simulink model "QBot2_TRIAL_1"  (Simulink 8.6)
settings: Solver=ode1  StartTime=0.0  StopTime=inf  FixedStep=0.01  RelTol=1e-3
undefined symbols (not defined in the file): HIL, Kinect, qc_get_step_size
libraries: quarc_library x13, simulink x1
settings Model: Creator=drmadill  LastModifiedBy=rclue  SimulationMode=external  ExtModeTrigDuration=1
settings SolverCC: PositivePriorityOrder=on
settings DebuggingCC: FcnCallInpInsideContextMsg=UseLocalSettings
settings RTWCC: SystemTargetFile=quarc_linux_duovero.tlc  TemplateMakefile=quarc_linux_duovero_tmf  Description=QUARC Linux DuoVero Target
settings STFCustomTargetCC: TargetLibSuffix=.a  TargetPreCompLibLocation=C:\PROGRA~3\QUARC\lib\2015b\LINUX_~1\release  ConcurrentExecutionCompliant=on  GeneratePreprocessorConditionals=Disable all  CPPClassGenCompliant=on  SystemTargetFile=quarc_linux_duovero.tlc
settings GRTTargetCC: TargetLibSuffix=.a  TargetPreCompLibLocation=C:\PROGRA~3\QUARC\lib\2015b\LINUX_~1\release  ParMdlRefBuildCompliant=off  CompOptLevelCompliant=off  MatFileLogging=off  UseToolchainInfoCompliant=off  ExtMode=on  ExtModeMexFile=quarc_comm  ExtModeMexArgs='-w -d /tmp -uri %u', 'tcpip://192.168.2.49:17001'

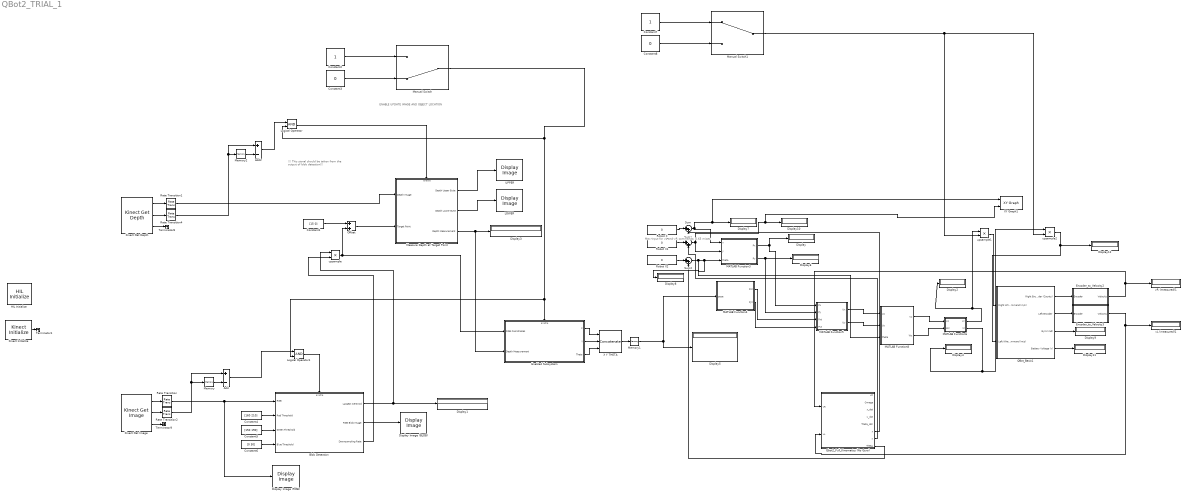
== system QBot2_TRIAL_1 ==
  note: ENABLE UPDATE IMAGE AND OBJECT LOCATION
  note: !!! This signal should be taken from the output of blob detection!!!
  note: Max input for vL and vR commands: 0.65 m/sec
  Add : Sum  Inputs=+-
  Add2 : Sum  Inputs=+-
  Blob Detection : Subsystem  TreatAsAtomicUnit=on
  Constant1 : Constant  Value=[15 0]
  Constant2 : Constant
  Constant3 : Constant  Value=0
  Constant4 : Constant  Value=[160 210]
  Constant5 : Constant  Value=[150 190]
  Constant6 : Constant  Value=[0 30]
  Constant7 : Constant
  Constant8 : Constant  Value=0
  Display{,1..12} (13 alike) : Display
  Display Image (BLOB) : quarc_library/Sinks/Figures/Display Image  figure_mode=Use figure window  figure_tag=figure1  axes_tag=axes1  update_rate=1  initial_position="167  215  854  628"  initial_visibility=off  sample_time=-1  axes_only=off  orig_size=off
  Display Image (RGB) : quarc_library/Sinks/Figures/Display Image  figure_mode=Use figure window  figure_tag=figure1  axes_tag=axes1  update_rate=1  initial_position="328  208  854  628"  initial_visibility=off  sample_time=-1  axes_only=off  orig_size=off
  Enabled Subsystem : Subsystem  TreatAsAtomicUnit=on
  Encoder_to_Velocity2 : Subsystem
  Encoder_to_Velocity3 : Subsystem
  HIL Initialize : quarc_library/Data Acquisition/Generic/Configuration/HIL Initialize  Priority=-99  object_name=HIL-1  board_type=qbot2  board_number=0  board_options=enc0_dir=0;enc0_filter=1;enc0_a=0;enc0_b=0;enc0_z=1;enc0_reload=0;enc1_dir=0;enc1_filter=1;enc1_a=0;enc1_b=0;enc1_z=1;enc1_reload=0;pwm0_immediate=0;pwm1_immediate=0;pwm2_immediate=0;pwm3_immediate=0;  exclusive=off  active=off  hardware_clocks=[]  clock_modes=[]  initial_clock_frequencies=[]  set_clock_params_at_start=off  set_clock_params_at_switch_in=off  set_clock_frequencies_at_start=off  set_clock_frequencies_at_switch_in=off  analog_input_channels=[0:9]  analog_input_maximums=[5 5 5 5 16.5 3.3 3.3 3.3 3.3]  analog_input_minimums=[0 0 0 0 0 0 0 0 0]  set_analog_input_params_at_start=off  set_analog_input_params_at_switch_in=off  analog_output_channels=[]  analog_output_maximums=[]  analog_output_minimums=[]  initial_analog_outputs=[]  final_analog_outputs=[]  watchdog_analog_outputs=[]  set_analog_output_params_at_start=off  set_analog_output_params_at_switch_in=off  set_analog_outputs_at_start=off  set_analog_outputs_at_switch_in=off  set_analog_outputs_at_terminate=off  set_analog_outputs_at_switch_out=off  set_analog_outputs_on_watchdog=off  digital_input_channels=[]  digital_output_channels=[]  digital_output_configuration=[]  initial_digital_outputs=[0]  final_digital_outputs=[0]  watchdog_digital_outputs=[0]  set_digital_output_params_at_start=off  set_digital_output_params_at_switch_in=off  set_digital_outputs_at_start=on  set_digital_outputs_at_switch_in=off  set_digital_outputs_at_terminate=on  set_digital_outputs_at_switch_out=off  set_digital_outputs_on_watchdog=on  encoder_channels=[0:3]  quadrature=[4]  encoder_filter_frequency=[]  initial_encoder_counts=[0]  set_encoder_params_at_start=on  set_encoder_params_at_switch_in=off  set_encoder_counts_at_start=on  set_encoder_counts_at_switch_in=off  pwm_channels=[0:3]  pwm_modes=[0]  pwm_frequency=[20e6/1024]  pwm_configuration=[0]  pwm_alignment=[0]  pwm_polarity=[1]  pwm_leading_deadband=[0]  pwm_trailing_deadband=[0]  initial_pwm_outputs=[0]  final_pwm_outputs=[0]  watchdog_pwm_outputs=[0]  set_pwm_params_at_start=on  set_pwm_params_at_switch_in=off  set_pwm_outputs_at_start=on  set_pwm_outputs_at_switch_in=off  set_pwm_outputs_at_terminate=on  set_pwm_outputs_at_switch_out=off  set_pwm_outputs_on_watchdog=on  other_output_channels=[2000:2001 14000 16000]  initial_other_outputs=[0 0 0 7]  final_other_outputs=[0 0 0 7]  watchdog_other_outputs=[]  set_other_outputs_at_start=on  set_other_outputs_at_switch_in=off  set_other_outputs_at_terminate=on  set_other_outputs_at_switch_out=off  set_other_outputs_on_watchdog=off
  Kinect Get Depth : quarc_library/Multimedia/Kinect Get Depth  object_name=Kinect-1  resolution=640 x 480  sample_time=qc_get_step_size * ceil(0.1 / qc_get_step_size)  show_player=off
  Kinect Get Image : quarc_library/Multimedia/Kinect Get Image  object_name=Kinect-1  sensor_type=color  resolution=640 x 480  output_format=MATLAB RGB (HxWx3)  data_type=uint8  backlight=average brightness  flicker=none  brightness=0.2156  gain=1.0  gamma=2.2  autoexposure=on  exposure=0  contrast=1.0  sharpness=0.5  hue=0.0  saturation=1.0  autobalance=on  balance=2700  frame_interval=0  sample_time=qc_get_step_size * ceil(0.1 / qc_get_step_size)
  Kinect Initialize : quarc_library/Multimedia/Kinect Initialize  object_name=Kinect-1  kinect_type=Kinect for XBox 360  identifier=0  sample_time=qc_get_step_size * ceil(0.033 / qc_get_step_size)  active=on
  LOWER : quarc_library/Sinks/Figures/Display Image  figure_mode=Use figure window  figure_tag=figure1  axes_tag=axes1  update_rate=1  initial_position="340  252  854  628"  initial_visibility=off  sample_time=-1  axes_only=off  orig_size=off
  Logical Operator : Logic  AllPortsSameDT=off  OutDataTypeStr=boolean
  Logical Operator1 : Logic  AllPortsSameDT=off  OutDataTypeStr=boolean
  MATLAB Function3 : MATLAB Function  TreatAsAtomicUnit=on
  MATLAB Function4 : MATLAB Function  TreatAsAtomicUnit=on
  MATLAB Function5 : MATLAB Function  TreatAsAtomicUnit=on
  MATLAB Function6 : MATLAB Function  TreatAsAtomicUnit=on
  MATLAB Function8 : MATLAB Function  TreatAsAtomicUnit=on
  Manual Switch : ManualSwitch  CurrentSetting=0
  Manual Switch1 : ManualSwitch
  Measure Depth at Target Point : Subsystem  TreatAsAtomicUnit=on
  Memory : Memory
  Memory1 : Memory
  Memory2 : Memory
  Offset : Sum
  QBot_Basic1 : Subsystem
  Qbot2_Full_Kinematics (No Gyro) : Subsystem
  Rate Transition{,1..2,4} (4 alike) : RateTransition
  Robot X : Constant  Value=0
  Robot X1 : Constant  Value=0
  Robot X2 : Constant  Value=0
  Sum : Sum  Inputs=|++
  Sum1 : Sum  Inputs=|++
  Sum2 : Sum  Inputs=|++
  Terminator1 : Terminator
  Terminator8 : Terminator
  Terminator9 : Terminator
  UPPER : quarc_library/Sinks/Figures/Display Image  figure_mode=Use figure window  figure_tag=figure1  axes_tag=axes1  update_rate=1  initial_position="188  236  854  628"  initial_visibility=off  sample_time=-1  axes_only=off  orig_size=off
  X Y THETA : Concatenate  NumInputs=3  ConcatenateDimension=3
  XY Graph1 : simulink/Sinks/XY Graph  xmin=-3  xmax=3  ymin=-3  ymax=3  st=-1
  upsample : Product
  upsample1 : Product
  upsample2 : Product
  vL (measured)1 : Display
  vR (measured)1 : Display
  wires:
  Kinect Initialize/1 -> Terminator1/1
  Rate Transition4/1 -> Add2/1, Memory2/1
  Memory2/1 -> Add2/2
  Kinect Get Depth/1 -> Rate Transition1/1
  Kinect Get Depth/2 -> Rate Transition4/1
  Kinect Get Depth/3 -> Terminator8/1
  Constant4/1 -> Blob Detection/2(Red Threshold)
  Constant5/1 -> Blob Detection/3(Green Threshold)
  Constant6/1 -> Blob Detection/4(Blue Threshold)
  Kinect Get Image/1 -> Rate Transition/1
  Kinect Get Image/2 -> Rate Transition2/1
  Rate Transition2/1 -> Add/1, Memory/1
  Kinect Get Image/3 -> Terminator9/1
  Rate Transition/1 -> Display Image (RGB)/1, Blob Detection/1(RGB)
  Blob Detection/2(RGB Blob Image) -> Display Image (BLOB)/1
  Rate Transition1/1 -> Measure Depth at Target Point/1(Depth Image)
  Constant1/1 -> Offset/1
  Measure Depth at Target Point/3(Depth Measurement) -> Enabled Subsystem/2(Depth Measurement), Display3/1
  Blob Detection/1(Largest Centroid) -> upsample/1, Display1/1
  Blob Detection/3(Downsampling Rate) -> upsample/2
  Measure Depth at Target Point/1(Depth Upper Byte) -> UPPER/1
  Measure Depth at Target Point/2(Depth Lower Byte) -> LOWER/1
  Offset/1 -> Measure Depth at Target Point/2(Target Point)
  Memory/1 -> Add/2
  MATLAB Function4/1(Pxt) -> MATLAB Function5/3(Pxt)
  MATLAB Function4/2(Pyt) -> MATLAB Function5/4(Pyt)
  MATLAB Function3/2(Py) -> MATLAB Function5/2(Py), Display6/1
  MATLAB Function3/1(Px) -> MATLAB Function5/1(Px), Display/1
  Sum2/1 -> MATLAB Function8/3(theta), Display8/1, MATLAB Function3/3(theta)
  Robot X2/1 -> Sum2/1
  Robot X/1 -> Sum/1
  Robot X1/1 -> Sum1/1
  MATLAB Function5/1(Ux) -> MATLAB Function8/1(Ux)
  MATLAB Function5/2(Uy) -> MATLAB Function8/2(Uy)
  MATLAB Function8/1(Vc) -> MATLAB Function6/1(Vc)
  MATLAB Function8/2(Wc) -> MATLAB Function6/2(Wc)
  MATLAB Function6/1(Vr) -> upsample1/1, Display2/1
  MATLAB Function6/2(Vl) -> Display4/1, upsample2/1
  QBot_Basic1/1(Right Encoder (Counts)) -> Encoder_to_Velocity2/1(Encoder)
  QBot_Basic1/2(Left Encoder) -> Encoder_to_Velocity3/1(Encoder)
  QBot_Basic1/3(Gyro (rad)) -> Display9/1
  QBot_Basic1/4(Battery Voltage (v)) -> Display11/1
  Encoder_to_Velocity2/1(Velocity) -> Qbot2_Full_Kinematics (No Gyro)/1(vR), vR (measured)1/1
  Encoder_to_Velocity3/1(Velocity) -> Qbot2_Full_Kinematics (No Gyro)/2(vL), vL (measured)1/1
  Sum1/1 -> MATLAB Function3/2(y), XY Graph1/2, Display10/1
  Sum/1 -> MATLAB Function3/1(x), XY Graph1/1, Display7/1
  Qbot2_Full_Kinematics (No Gyro)/6(x) -> Sum/2
  Qbot2_Full_Kinematics (No Gyro)/7(y) -> Sum1/2
  Qbot2_Full_Kinematics (No Gyro)/8(Theta) -> Sum2/2
  upsample/1 -> Offset/2, Enabled Subsystem/1(RGB Coordinates)
  Enabled Subsystem/2(Y) -> X Y THETA/2
  Enabled Subsystem/1(X) -> X Y THETA/1
  Enabled Subsystem/3(Theta) -> X Y THETA/3
  Constant3/1 -> Manual Switch/2
  Constant2/1 -> Manual Switch/1
  Manual Switch/1 -> Logical Operator/2, Logical Operator1/2, Enabled Subsystem/Enable
  X Y THETA/1 -> Memory1/1
  Memory1/1 -> MATLAB Function4/1(pose), Display5/1
  upsample1/1 -> QBot_Basic1/1(Right Wheel Command (m/s))
  upsample2/1 -> Display12/1, QBot_Basic1/2(Left Wheel Command (m/s))
  Constant8/1 -> Manual Switch1/2
  Constant7/1 -> Manual Switch1/1
  Manual Switch1/1 -> upsample2/2, upsample1/2
  Add2/1 -> Logical Operator/1
  Add/1 -> Logical Operator1/1
  Logical Operator1/1 -> Blob Detection/Enable
  Logical Operator/1 -> Measure Depth at Target Point/Enable

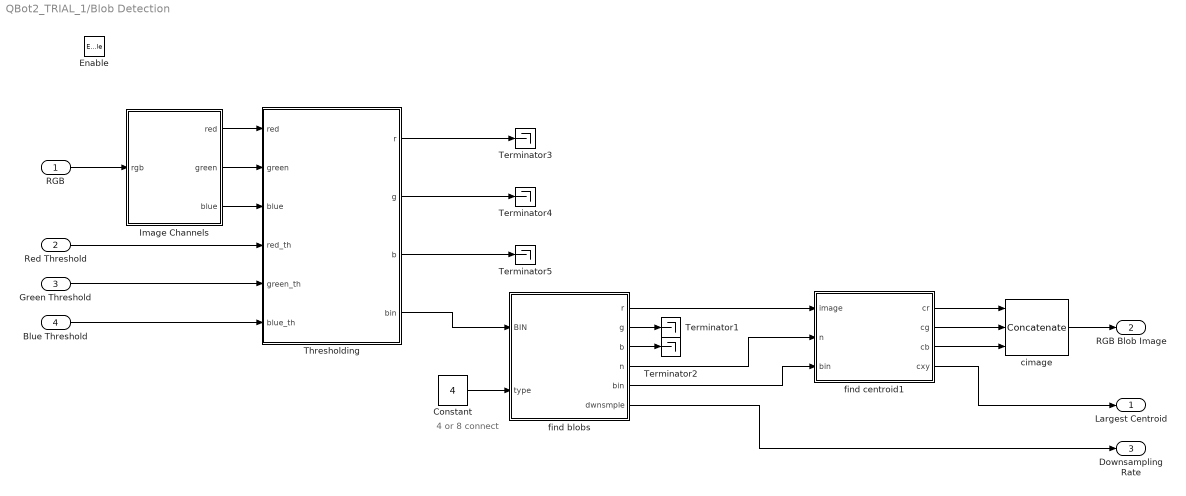
== system QBot2_TRIAL_1/Blob Detection ==
  note: 4 or 8 connect
  RGB : Inport
  Red Threshold : Inport  Port=2
  Green Threshold : Inport  Port=3
  Blue Threshold : Inport  Port=4
  Enable : EnablePort
  Constant : Constant  Value=4
  Image Channels : Subsystem
  Terminator{1..5} (5 alike) : Terminator
  Thresholding : MATLAB Function  TreatAsAtomicUnit=on
  cimage : Concatenate  NumInputs=3  Mode=Multidimensional array  ConcatenateDimension=3
  find blobs : MATLAB Function  TreatAsAtomicUnit=on
  find centroid1 : MATLAB Function  TreatAsAtomicUnit=on
  Largest Centroid : Outport
  RGB Blob Image : Outport  Port=2
  Downsampling Rate : Outport  Port=3
  wires:
  Image Channels/1(red) -> Thresholding/1(red)
  Image Channels/2(green) -> Thresholding/2(green)
  Image Channels/3(blue) -> Thresholding/3(blue)
  Thresholding/4(bin) -> find blobs/1(BIN)
  RGB/1 -> Image Channels/1(rgb)
  Blue Threshold/1 -> Thresholding/6(blue_th)
  Green Threshold/1 -> Thresholding/5(green_th)
  Red Threshold/1 -> Thresholding/4(red_th)
  Constant/1 -> find blobs/2(type)
  find blobs/2(g) -> Terminator1/1
  find blobs/3(b) -> Terminator2/1
  find blobs/1(r) -> find centroid1/1(image)
  find blobs/4(n) -> find centroid1/2(n)
  find centroid1/4(cxy) -> Largest Centroid/1
  find centroid1/1(cr) -> cimage/1
  find centroid1/2(cg) -> cimage/2
  find centroid1/3(cb) -> cimage/3
  cimage/1 -> RGB Blob Image/1
  Thresholding/1(r) -> Terminator3/1
  Thresholding/2(g) -> Terminator4/1
  Thresholding/3(b) -> Terminator5/1
  find blobs/6(dwnsmple) -> Downsampling Rate/1
  find blobs/5(bin) -> find centroid1/3(bin)

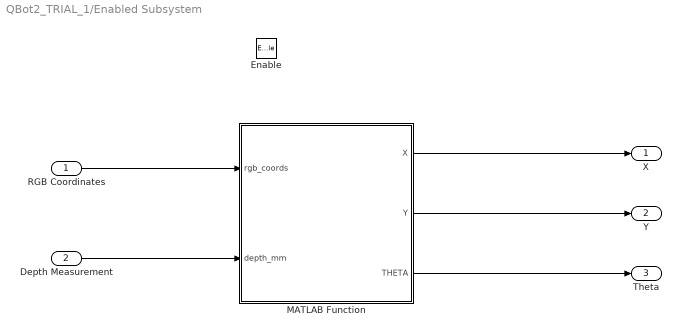
== system QBot2_TRIAL_1/Enabled Subsystem ==
  RGB Coordinates : Inport
  Depth Measurement : Inport  Port=2
  Enable : EnablePort
  MATLAB Function : MATLAB Function  TreatAsAtomicUnit=on
  X : Outport
  Y : Outport  Port=2
  Theta : Outport  Port=3
  wires:
  RGB Coordinates/1 -> MATLAB Function/1(rgb_coords)
  Depth Measurement/1 -> MATLAB Function/2(depth_mm)
  MATLAB Function/1(X) -> X/1
  MATLAB Function/2(Y) -> Y/1
  MATLAB Function/3(THETA) -> Theta/1

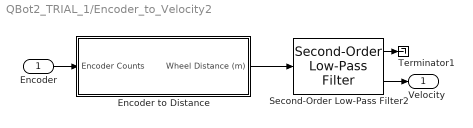
== system QBot2_TRIAL_1/Encoder_to_Velocity2 ==
  Encoder : Inport
  Encoder to Distance : Subsystem
  Second-Order Low-Pass Filter2 : quarc_library/Continuous/Second-Order Low-Pass Filter  params_source=Internal (dialog parameters)  input_width=10  input_zeta=1  input_init=0
  Terminator1 : Terminator
  Velocity : Outport
  wires:
  Second-Order Low-Pass Filter2/2 -> Velocity/1
  Encoder/1 -> Encoder to Distance/1(Encoder Counts)
  Encoder to Distance/1(Wheel Distance (m)) -> Second-Order Low-Pass Filter2/1
  Second-Order Low-Pass Filter2/1 -> Terminator1/1

== system QBot2_TRIAL_1/Encoder_to_Velocity3 ==
  Encoder : Inport
  Encoder to Distance : Subsystem
  Second-Order Low-Pass Filter2 : quarc_library/Continuous/Second-Order Low-Pass Filter  params_source=Internal (dialog parameters)  input_width=10  input_zeta=1  input_init=0
  Terminator1 : Terminator
  Velocity : Outport
  wires:
  Second-Order Low-Pass Filter2/2 -> Velocity/1
  Encoder/1 -> Encoder to Distance/1(Encoder Counts)
  Encoder to Distance/1(Wheel Distance (m)) -> Second-Order Low-Pass Filter2/1
  Second-Order Low-Pass Filter2/1 -> Terminator1/1

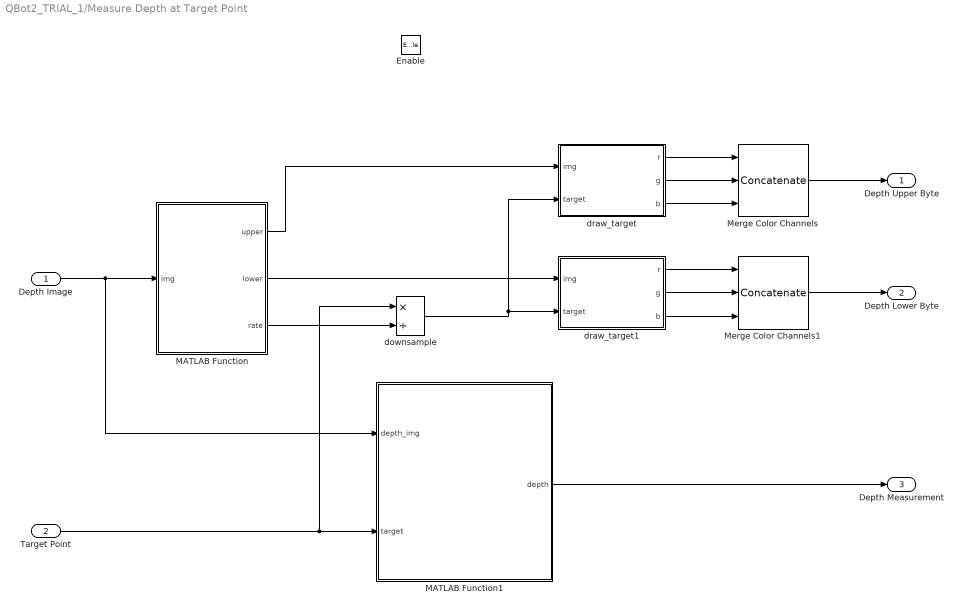
== system QBot2_TRIAL_1/Measure Depth at Target Point ==
  Depth Image : Inport
  Target Point : Inport  Port=2
  Enable : EnablePort
  MATLAB Function : MATLAB Function  TreatAsAtomicUnit=on
  MATLAB Function1 : MATLAB Function  TreatAsAtomicUnit=on
  Merge Color Channels : Concatenate  NumInputs=3  Mode=Multidimensional array  ConcatenateDimension=3
  Merge Color Channels1 : Concatenate  NumInputs=3  Mode=Multidimensional array  ConcatenateDimension=3
  downsample : Product  Inputs=*/
  draw_target : MATLAB Function  TreatAsAtomicUnit=on
  draw_target1 : MATLAB Function  TreatAsAtomicUnit=on
  Depth Upper Byte : Outport
  Depth Lower Byte : Outport  Port=2
  Depth Measurement : Outport  Port=3
  wires:
  Merge Color Channels/1 -> Depth Upper Byte/1
  Depth Image/1 -> MATLAB Function1/1(depth_img), MATLAB Function/1(img)
  draw_target/1(r) -> Merge Color Channels/1
  draw_target1/1(r) -> Merge Color Channels1/1
  draw_target/2(g) -> Merge Color Channels/2
  draw_target/3(b) -> Merge Color Channels/3
  draw_target1/2(g) -> Merge Color Channels1/2
  draw_target1/3(b) -> Merge Color Channels1/3
  Target Point/1 -> downsample/1, MATLAB Function1/2(target)
  Merge Color Channels1/1 -> Depth Lower Byte/1
  downsample/1 -> draw_target/2(target), draw_target1/2(target)
  MATLAB Function/1(upper) -> draw_target/1(img)
  MATLAB Function/2(lower) -> draw_target1/1(img)
  MATLAB Function/3(rate) -> downsample/2
  MATLAB Function1/1(depth) -> Depth Measurement/1

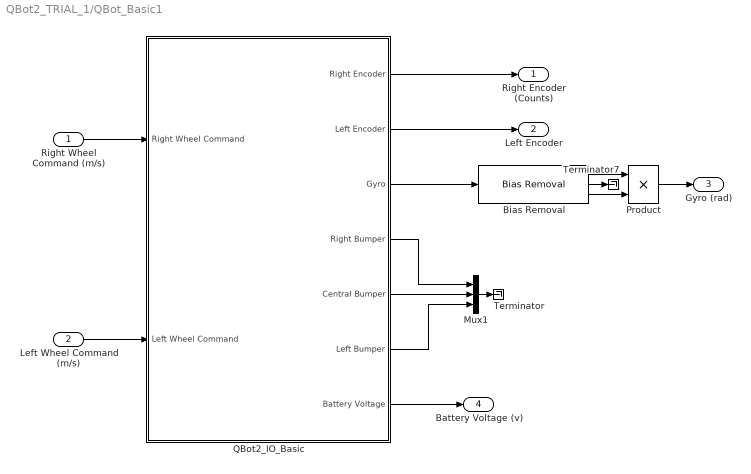
== system QBot2_TRIAL_1/QBot_Basic1 ==
  Right Wheel Command (m/s) : Inport
  Left Wheel Command (m/s) : Inport  Port=2
  Bias Removal : quarc_library/Discrete/Bias Removal  start_time=3  end_time=4  switch_id=0  sample_time=qc_get_step_size
  Mux1 : Mux  Inputs=3
  Product : Product  RndMeth=Zero
  QBot2_IO_Basic : Subsystem
  Terminator : Terminator
  Terminator7 : Terminator
  Right Encoder (Counts) : Outport
  Left Encoder : Outport  Port=2
  Gyro (rad) : Outport  Port=3
  Battery Voltage (v) : Outport  Port=4
  wires:
  Mux1/1 -> Terminator/1
  QBot2_IO_Basic/3(Gyro) -> Bias Removal/1
  Product/1 -> Gyro (rad)/1
  Bias Removal/3 -> Product/2
  Bias Removal/1 -> Product/1
  Bias Removal/2 -> Terminator7/1
  QBot2_IO_Basic/7(Battery Voltage) -> Battery Voltage (v)/1
  QBot2_IO_Basic/2(Left Encoder) -> Left Encoder/1
  QBot2_IO_Basic/1(Right Encoder) -> Right Encoder (Counts)/1
  Left Wheel Command (m/s)/1 -> QBot2_IO_Basic/2(Left Wheel Command)
  Right Wheel Command (m/s)/1 -> QBot2_IO_Basic/1(Right Wheel Command)
  QBot2_IO_Basic/6(Left Bumper) -> Mux1/3
  QBot2_IO_Basic/5(Central Bumper) -> Mux1/2
  QBot2_IO_Basic/4(Right Bumper) -> Mux1/1

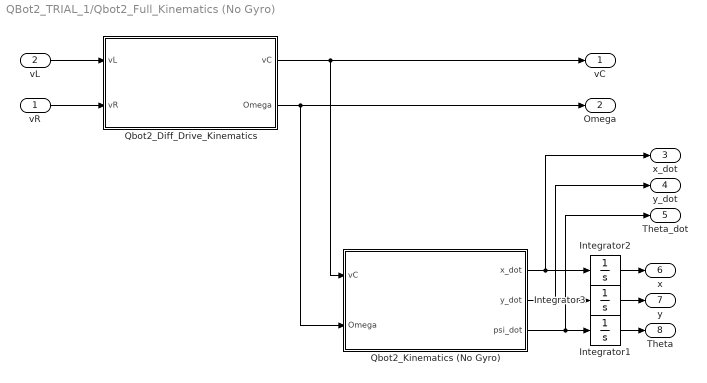
== system QBot2_TRIAL_1/Qbot2_Full_Kinematics (No Gyro) ==
  vR : Inport
  vL : Inport  Port=2
  Integrator1 : Integrator
  Integrator2 : Integrator
  Integrator3 : Integrator
  Qbot2_Diff_Drive_Kinematics : Subsystem
  Qbot2_Kinematics (No Gyro) : Subsystem
  vC : Outport
  Omega : Outport  Port=2
  x_dot : Outport  Port=3
  y_dot : Outport  Port=4
  Theta_dot : Outport  Port=5
  x : Outport  Port=6
  y : Outport  Port=7
  Theta : Outport  Port=8
  wires:
  Qbot2_Diff_Drive_Kinematics/2(Omega) -> Omega/1, Qbot2_Kinematics (No Gyro)/2(Omega)
  Integrator3/1 -> y/1
  Integrator2/1 -> x/1
  vR/1 -> Qbot2_Diff_Drive_Kinematics/2(vR)
  vL/1 -> Qbot2_Diff_Drive_Kinematics/1(vL)
  Qbot2_Diff_Drive_Kinematics/1(vC) -> vC/1, Qbot2_Kinematics (No Gyro)/1(vC)
  Qbot2_Kinematics (No Gyro)/2(y_dot) -> Integrator3/1, y_dot/1
  Qbot2_Kinematics (No Gyro)/1(x_dot) -> Integrator2/1, x_dot/1
  Qbot2_Kinematics (No Gyro)/3(psi_dot) -> Integrator1/1, Theta_dot/1
  Integrator1/1 -> Theta/1

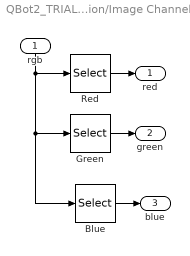
== system QBot2_TRIAL_1/Blob Detection/Image Channels ==
  rgb : Inport
  Blue : Selector  NumberOfDimensions=3  InputPortWidth=3  IndexOptions=Select all,Select all,Index vector (dialog)  Indices=1,1,3  OutputSizes=1,1,1
  Green : Selector  NumberOfDimensions=3  InputPortWidth=3  IndexOptions=Select all,Select all,Index vector (dialog)  Indices=1,1,2  OutputSizes=1,1,1
  Red : Selector  NumberOfDimensions=3  InputPortWidth=3  IndexOptions=Select all,Select all,Index vector (dialog)  Indices=[1 3],1,1  OutputSizes=1,1,1
  red : Outport
  green : Outport  Port=2
  blue : Outport  Port=3
  wires:
  rgb/1 -> Red/1, Blue/1, Green/1
  Red/1 -> red/1
  Green/1 -> green/1
  Blue/1 -> blue/1

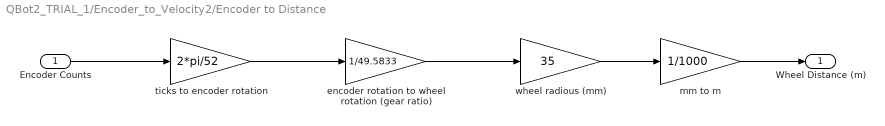
== system QBot2_TRIAL_1/Encoder_to_Velocity2/Encoder to Distance ==
  Encoder Counts : Inport
  " encoder rotation to wheel rotation (gear ratio)" : Gain  Gain=1/49.5833
  mm to m : Gain  Gain=1/1000
  ticks to encoder rotation : Gain  Gain=2*pi/52
  wheel radious (mm) : Gain  Gain=35
  Wheel Distance (m) : Outport
  wires:
  mm to m/1 -> Wheel Distance (m)/1
  wheel radious (mm)/1 -> mm to m/1
  " encoder rotation to wheel rotation (gear ratio)"/1 -> wheel radious (mm)/1
  ticks to encoder rotation/1 -> " encoder rotation to wheel rotation (gear ratio)"/1
  Encoder Counts/1 -> ticks to encoder rotation/1

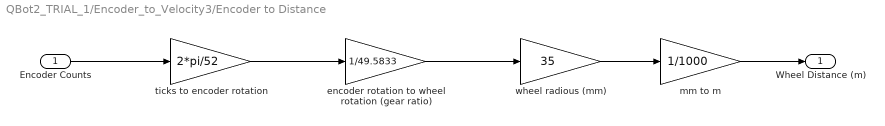
== system QBot2_TRIAL_1/Encoder_to_Velocity3/Encoder to Distance ==
  Encoder Counts : Inport
  " encoder rotation to wheel rotation (gear ratio)" : Gain  Gain=1/49.5833
  mm to m : Gain  Gain=1/1000
  ticks to encoder rotation : Gain  Gain=2*pi/52
  wheel radious (mm) : Gain  Gain=35
  Wheel Distance (m) : Outport
  wires:
  mm to m/1 -> Wheel Distance (m)/1
  wheel radious (mm)/1 -> mm to m/1
  " encoder rotation to wheel rotation (gear ratio)"/1 -> wheel radious (mm)/1
  ticks to encoder rotation/1 -> " encoder rotation to wheel rotation (gear ratio)"/1
  Encoder Counts/1 -> ticks to encoder rotation/1

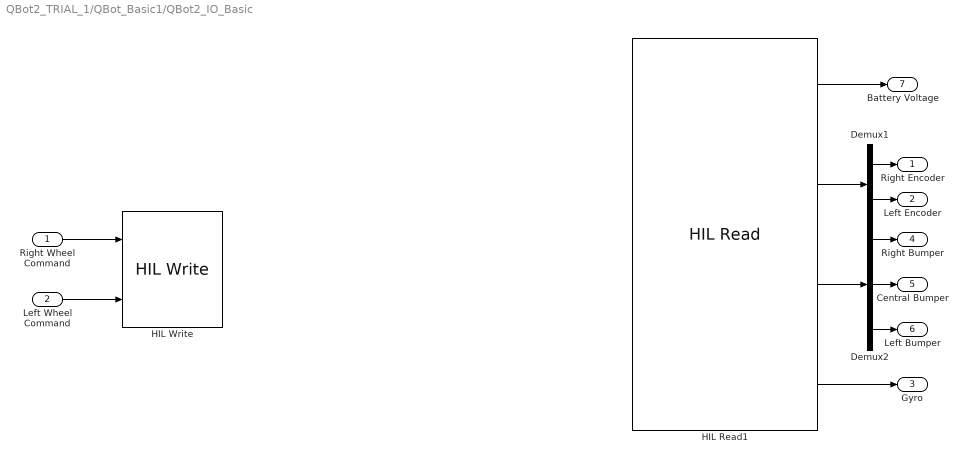
== system QBot2_TRIAL_1/QBot_Basic1/QBot2_IO_Basic ==
  Right Wheel Command : Inport
  Left Wheel Command : Inport  Port=2
  Demux1 : Demux  Outputs=2
  Demux2 : Demux  Outputs=3
  HIL Read1 : quarc_library/Data Acquisition/Generic/Immediate I//O/HIL Read  object_name=HIL-1  analog_channels=[4]  encoder_channels=[2 3]  digital_channels=[8 9 10]  other_channels=[1002]  sample_time=qc_get_step_size  active=on  vector_output=on  data_type_mode=Inherit via back propagation  encoder_data_type=double  digital_data_type=boolean
  HIL Write : quarc_library/Data Acquisition/Generic/Immediate I//O/HIL Write  object_name=HIL-1  analog_channels=[]  pwm_channels=[]  digital_channels=[]  other_channels=[2000:2001]  sample_time=-1  active=on  vector_input=off
  Right Encoder : Outport
  Left Encoder : Outport  Port=2
  Gyro : Outport  Port=3
  Right Bumper : Outport  Port=4
  Central Bumper : Outport  Port=5
  Left Bumper : Outport  Port=6
  Battery Voltage : Outport  Port=7
  wires:
  Demux2/3 -> Left Bumper/1
  Demux2/2 -> Central Bumper/1
  Demux2/1 -> Right Bumper/1
  HIL Read1/2 -> Demux1/1
  Left Wheel Command/1 -> HIL Write/2
  Right Wheel Command/1 -> HIL Write/1
  Demux1/2 -> Left Encoder/1
  Demux1/1 -> Right Encoder/1
  HIL Read1/4 -> Gyro/1
  HIL Read1/3 -> Demux2/1
  HIL Read1/1 -> Battery Voltage/1

== system QBot2_TRIAL_1/Qbot2_Full_Kinematics (No Gyro)/Qbot2_Diff_Drive_Kinematics ==
  vL : Inport
  vR : Inport  Port=2
  Qbot2_Diff_Drive_Kinematics : MATLAB Function  TreatAsAtomicUnit=on
  vC : Outport
  Omega : Outport  Port=2
  wires:
  Qbot2_Diff_Drive_Kinematics/2(Omega) -> Omega/1
  vR/1 -> Qbot2_Diff_Drive_Kinematics/2(vR)
  Qbot2_Diff_Drive_Kinematics/1(vC) -> vC/1
  vL/1 -> Qbot2_Diff_Drive_Kinematics/1(vL)

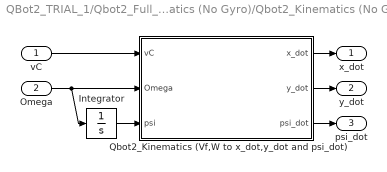
== system QBot2_TRIAL_1/Qbot2_Full_Kinematics (No Gyro)/Qbot2_Kinematics (No Gyro) ==
  vC : Inport
  Omega : Inport  Port=2
  Integrator : Integrator
  Qbot2_Kinematics (Vf,W to x_dot,y_dot and psi_dot) : MATLAB Function  TreatAsAtomicUnit=on
  x_dot : Outport
  y_dot : Outport  Port=2
  psi_dot : Outport  Port=3
  wires:
  Qbot2_Kinematics (Vf,W to x_dot,y_dot and psi_dot)/2(y_dot) -> y_dot/1
  Omega/1 -> Qbot2_Kinematics (Vf,W to x_dot,y_dot and psi_dot)/2(Omega), Integrator/1
  Qbot2_Kinematics (Vf,W to x_dot,y_dot and psi_dot)/1(x_dot) -> x_dot/1
  vC/1 -> Qbot2_Kinematics (Vf,W to x_dot,y_dot and psi_dot)/1(vC)
  Integrator/1 -> Qbot2_Kinematics (Vf,W to x_dot,y_dot and psi_dot)/3(psi)
  Qbot2_Kinematics (Vf,W to x_dot,y_dot and psi_dot)/3(psi_dot) -> psi_dot/1

== matlab function Measure Depth at Target Point/MATLAB Function ==
  data: img input double; upper output double; lower output double; rate output double
function [upper, lower, rate]   = downsample(img)
%#codegen

%constants
rate = 2;
offset = rate/2;
new_row = 480/rate;
new_col = 640/rate;


% The Kinect depth sensor range is: minimum 800mm and maximum 4000mm. 
% The Kinect for Windows Hardware can however be switched to Near Mode 
% which provides a range of 500mm to 3000mm instead of the Default range


lower = uint8(zeros(new_row, new_col));
upper = uint8(zeros(new_row, new_col));


u = offset;
v = offset;
for i=1:new_row
    for j=1:new_col

        lower(i,j) = uint8(mod(img(u,v), 256));
        upper(i,j) = uint8(bitshift(img(u,v), -8)); 
        % NOTE: img(u,v) / 256 does not produce correct measurement for
        % some distances (90 cm for us)
        
        
        v = v + rate;
    end
    
    v = offset;
    u = u + rate;
end

== matlab function Blob Detection/Thresholding ==
  data: red input double; r output double; g output double; b output double; bin output double; green input double; blue input double; red_th input double; green_th input double; blue_th input double
function [r, g, b, bin]  = clr_thr(red, ...
    green, blue, red_th, green_th, blue_th)
% This block supports the Embedded MATLAB subset.
% See the help menu for details. 

red_vec = thresh(red, red_th, 1);

green_vec = thresh(green, green_th, 1);

blue_vec = thresh(blue, blue_th, 1);

tmp = double(and(red_vec, green_vec));
tmp_blob = uint8(and(tmp, blue_vec));
bin = uint8(255*tmp_blob);

% background = uint8(255*double(not(tmp_blob)));
% r = uint8(red.*tmp_blob + background);
% g = uint8(green.*tmp_blob + background);
% b = uint8(blue.*tmp_blob + background);

r = uint8(red.*tmp_blob);
g = uint8(green.*tmp_blob);
b = uint8(blue.*tmp_blob);


return;

%--------------------------------------------------------------------------

function x = thresh(x, th, val)

[row col] = size(x);
for i=1:row
    for j=1:col
        if x(i,j) >= th(1) && x(i, j) <= th(2)
            x(i, j) = val;
        else
            x(i, j) = 0;
        end
    end
end

return;

%--------------------------------------------------------------------------

== matlab function MATLAB Function3 ==
  data: x input double; Px output double; Py output double; y input double; theta input double
function [Px,Py] = PxPy_convert(x, y, theta)

l=.0235; %#length between the two wheels in meters
%R=.0175; %#R or signed distance from ICC (Instanteous center of curvature) in meters
Px= x+l*cos(theta)
Py = y+l*sin(theta)

%#codegen

== matlab function MATLAB Function4 ==
  data: pose input double; Pxt output double; Pyt output double
function [Pxt,Pyt] = PxtPyt_convert(pose)
x=pose(1);
y=pose(2);
theta=pose(2);
l=.0235; %#length between the two wheels in meters
%R=.0175; %#R or signed distance from ICC (Instanteous center of curvature) in meters
Pxt= x+l*cos(theta)
Pyt = y+l*sin(theta)

%#codegen

== matlab function Blob Detection/find blobs ==
  data: BIN input double; r output double; g output double; b output double; n output double; bin output double; type input double; dwnsmple output double
function [r, g, b, n, bin, dwnsmple]  = find_blobs(BIN, type)
% This block supports the Embedded MATLAB subset.
% See the help menu for details. 

idvec = zeros(1, 50);

[ROW COL] = size(BIN);

%{
if ROW>120 || COL>160
    r = uint8(BIN);
    g = uint8(BIN);
    b = uint8(BIN);
    n = -1;
    return;
end
%}



dwnsmple = 2;
row = round(ROW/dwnsmple);
col = round(COL/dwnsmple);
bin = uint8(zeros(row, col));

rw = 0;
% for i=dwnsmple+1:dwnsmple:ROW
for i=1:dwnsmple:ROW
    rw = rw + 1;
    co = 0;
    for j=1:dwnsmple:COL
        co = co + 1;
        bin(rw, co) = uint8(BIN(i, j));
    end
end

% r = uint8(zeros(row, col));
% g = uint8(zeros(row, col));
% b = uint8(zeros(row, col));
r = uint8(bin);
g = uint8(bin);
b = uint8(bin);
n = -1;%count;

% Bin = double(bin)/255;
% binsum = sum(Bin(:));
% ratio = binsum/(row*col);

% if ratio<=0.1
    % Find the 4 or 8 connected reachability matrix
    [eqtable, limg, maxlabel] = find_reachability_matrix(bin, type);
    if maxlabel>=1
        % Find equivalent labels
        table1 = updatetable(eqtable, maxlabel);
        table2 = updatetable2(table1, maxlabel);
        table3 = double(or(table1, table2));
        [idvec, n] = updatetable3(table3, maxlabel);
%     
%     
%         % Label the final image
        Limg = label_image(limg, n, idvec, maxlabel);
        r = uint8(Limg);
        g = uint8(Limg);
        b = uint8(Limg);
    end
%     r = uint8(limg);
%     g = uint8(limg);
%     b = uint8(limg);
% end



return;
%--------------------------------------------------------------------------
function [eqtable, limg, maxlabel] = find_reachability_matrix(img, Type)

[row col] = size(img);

type = Type;
if Type~=4 && Type~=8
    type = 8;
end

% Step 1: Label 8 or 4 connected components
limg = zeros(row, col);
label = 0;
Maxlabel = 50;
for i=1:row
    for j=1:col
        if img(i, j)>0 && limg(i, j)==0
            if (j-1)>=1 && img(i, j-1)>0
                limg(i, j)= limg(i, j-1);
            else
                if label<=(Maxlabel-1)
                    label = label+1;
                    limg(i, j)= label;
                else
                    limg(i, j)= 0;
                end
            end
        end
    end
end

% Find the reachability matrix
maxlabel = label;
eqtable = eye(Maxlabel, Maxlabel);
if maxlabel<1
    return;
end
% eqtable = eye(maxlabel, maxlabel);
for i=2:row
    for j=1:col
        if type == 4
            if img(i, j)>0
                if img(i-1, j)>0 && limg(i, j)~=0
                    eqtable(limg(i, j), limg(i-1, j)) = 1;
                    eqtable(limg(i-1, j), limg(i, j)) = 1;
                end
            end
        elseif type == 8
            if img(i, j)>0 && limg(i, j)~=0
                if (j-1)>=1 && img(i-1, j-1)>0 
                    eqtable(limg(i, j), limg(i-1, j-1)) = 1;
                    eqtable(limg(i-1, j-1), limg(i, j)) = 1;
                end
                if img(i-1, j)>0
                    eqtable(limg(i, j), limg(i-1, j)) = 1;
                    eqtable(limg(i-1, j), limg(i, j)) = 1;
                end
                if (j+1)<=col && img(i-1, j+1)>0
                    eqtable(limg(i, j), limg(i-1, j+1)) = 1;
                    eqtable(limg(i-1, j+1), limg(i, j)) = 1;
                end
            end
        end
        
    end
end

return;
%--------------------------------------------------------------------------
function [table] = updatetable(eqtable, maxlabel)

[row col] = size(eqtable);
table = zeros(row, col);
% etable = eqtable;
for i=1:maxlabel
    tmp1 = eqtable(i, :);
    for j=i+1:maxlabel
        tmp2 = eqtable(j, :);
        iscommon = sum(double(and(tmp1, tmp2)));
        if iscommon
            tmp1 = double(or(tmp1, tmp2));
        end
    end
        table(i, :) = tmp1;
end

return;
%--------------------------------------------------------------------------
function [table] = updatetable2(eqtable, maxlabel)

[row col] = size(eqtable);
table = zeros(row, col);
% etable = eqtable;
for i=maxlabel:-1:1
    tmp1 = eqtable(i, :);
%         i
%         count = count + 1;
%         idvec(i) = count;
    for j=i-1:-1:1
        tmp2 = eqtable(j, :);
        iscommon = sum(double(and(tmp1, tmp2)));
        if iscommon
            tmp1 = double(or(tmp1, tmp2));
%                 find(tmp1==1)
%                 pause
        end
    end
    table(i, :) = tmp1;
end

return;
%--------------------------------------------------------------------------
function [idvec, count] = updatetable3(eqtable, maxlabel)

[row col] = size(eqtable);
table = zeros(row, col);
count = 0;
idvec = zeros(1, col);
% etable = eqtable;
for i=1:maxlabel
    tmp1 = eqtable(i, :);
    if tmp1(i)~=0
        count = count + 1;
        idvec(i) = count;
        for j=i+1:maxlabel
            tmp2 = eqtable(j, :);
            iscommon = sum(double(and(tmp1, tmp2)));
            if iscommon
                tmp1 = double(or(tmp1, tmp2));
            end
        end
        table(i, :) = tmp1;
        for j=i+1:maxlabel
            if tmp1(j)==1
                idvec(j) = count;
                eqtable(j, :) = table(j, :);
            end
        end
    end
end

return;
%--------------------------------------------------------------------------
function [Limg] = label_image(limg, count, idvec, maxlabel)

[row col] = size(limg);
Limg = limg;
for i=1:row
    for j=1:col
        if Limg(i, j)>0 && Limg(i, j)<=maxlabel
%             if count<=255
%                 Limg(i, j) = uint8(round((255/count)*idvec(Limg(i, j))));
%             else
                Limg(i, j) = uint8(idvec(Limg(i, j)));
%             end
        end
    end
end

return;
%--------------------------------------------------------------------------

== matlab function Blob Detection/find centroid1 ==
  data: cr output double; cg output double; cb output double; image input double; cxy output double; n input double; bin input double
function [cr, cg, cb, cxy]  = find_centroid(image, n, bin)
% This block supports the Embedded MATLAB subset.
% See the help menu for details. 


[binrow bincol] = size(bin);
cr = bin;
cg = bin;
cb = bin;
[row col] = size(image);
x = -1;
y = -1;
cxy = zeros(2,1);
if n>50
    cxy(1,1) = x;
    cxy(2,1) = y;
    return;
end
X = zeros(1, 50);
Y = zeros(1, 50);
N = zeros(1, 50);
for L=1:n
    for i=1:row
        for j=1:col
            if image(i, j) == L
                X(L) = X(L) + j;
                Y(L) = Y(L) + i;
                N(L) = N(L) + 1;
            end
        end
    end
end

maxN = -1;
maxNid = -1;
for L=1:n
    val = N(L);
    if val > maxN
        maxN = val;
        maxNid = L;
    end
end

if maxN > 0
    x = X(maxNid)/N(maxNid);
    y = Y(maxNid)/N(maxNid);
    
    for i=fix(y-2):fix(y+2)
        if i>=1 && i<=binrow
            for j=fix(x-2):fix(x+2) 
                if j>=1 && j<=bincol
                    cr(i, j) = 255;
                    cg(i, j) = 0;
                    cb(i, j) = 0;
                end
            end
        end
    end
    
end

cxy(1,1) = x;
cxy(2,1) = y;

return;
%--------------------------------------------------------------------------

== matlab function Measure Depth at Target Point/MATLAB Function1 ==
  data: depth_img input double; depth output double; target input double
function depth  = measure_pixel(depth_img, target)
%#codegen

x = target(1);
y = target(2);
[ymax, xmax] = size(depth_img);

depth = uint16(depth_img(y,x));

== matlab function Measure Depth at Target Point/draw_target ==
  data: img input double; r output double; target input double; g output double; b output double
function [r,g,b] = fcn(img, target)
%#codegen

tx = target(1);
ty = target(2);
[ymax, xmax] = size(img);
r = img;
g = img;
b = img;

if ty < ymax && ty > 1 && tx < xmax && tx > 1
    
    r(ty-1:ty+1,tx-1:tx+1) = 255;
    g(ty-1:ty+1,tx-1:tx+1) = 0;
    b(ty-1:ty+1,tx-1:tx+1) = 0;
end

== matlab function Measure Depth at Target Point/draw_target1 ==
  data: img input double; r output double; target input double; g output double; b output double
function [r,g,b] = fcn(img, target)
%#codegen

tx = target(1);
ty = target(2);
[ymax, xmax] = size(img);
r = img;
g = img;
b = img;

if ty < ymax && ty > 1 && tx < xmax && tx > 1
    
    r(ty-1:ty+1,tx-1:tx+1) = 255;
    g(ty-1:ty+1,tx-1:tx+1) = 0;
    b(ty-1:ty+1,tx-1:tx+1) = 0;
end

== matlab function MATLAB Function5 ==
  data: Px input double; Ux output double; Py input double; Pxt input double; Pyt input double; Uy output double
function [Ux, Uy] = UxUy(Px,Py,Pxt,Pyt)
%#codegen
%rho_star=.5;
%omega_star=.5;
 
krho = .75;
kphi = 1;
w_d=.05;
 
U = [0 0];
rho_size = .5;
phi_size = 1;
[phi, rho] = cart2pol(Px,Py);
[phi_d, rho_d] = cart2pol(Pxt,Pyt);
 
[phi_dif, rho_dif] = cart2pol((Px-Pxt),(Py-Pyt));
 
PxD = Px - Pxt; 
PyD = Py - Pyt;
 
 
 
J_i=[PxD/(sqrt(PxD^2+PyD^2)) PyD/(sqrt(PxD^2+PyD^2)); -PyD/(PxD^2+PyD^2) PxD/(PxD^2+PyD^2)];
 
 
 
 
%J_i=[(Px-Pxt)/phi_dif (Py-Pyt)/phi_dif;...
%    -(Py-Pyt)/((1+((Py-Pyt)/(PD))^2)*(Px-Pxt)^2)  1/((1+((Py-Pyt)/(PD))^2)*(Px-Pxt))];
 
 
 
%J_i=[ (Px-Pxt)/phi (Py-Pyt)/phi_dif;    -(Py-Pyt)/(phi_dif)^2  (Px-Pxt)/(phi_dif)^2 ];
 
rhoi_dot = krho*(rho_size-rho_dif)
%phii_d= phi/2
%phii_d = phi_d - phii_d
phii_dot = w_d; %+ kphi*((phi_size-phi)/2);
V_i= [rhoi_dot; phii_dot];
Rt = [ 1 0; 0 1];
 
 
U = Rt*(J_i'*V_i);
U = inv(J_i)*V_i; 
Ux = U(1);
Uy = U(2);

== matlab function MATLAB Function6 ==
  data: Vc input double; Vr output double; Wc input double; Vl output double
function [Vr,Vl] = VcWc2VrVl(Vc,Wc)
%#codegen

l=.0235;
Vr = Vc+(1/2)*(l*2)*Wc;
Vl = Vc-(1/2)*(l*2)*Wc;

== matlab function MATLAB Function8 ==
  data: Ux input double; Vc output double; Uy input double; Wc output double; theta input double
function [Vc,Wc] = UxUy2VcWc(Ux,Uy, theta)

l=.0235; %#length between the two wheels in meters
kin_inv = inv([cos(theta) -l*sin(theta) ; sin(theta) l*cos(theta)]);
P =  kin_inv*[Ux;Uy];
Vc=P(1);
Wc=P(2);

== matlab function Qbot2_Full_Kinematics (No Gyro)/Qbot2_Diff_Drive_Kinematics/Qbot2_Diff_Drive_Kinematics ==
  data: vL input double; vC output double; vR input double; Omega output double
function [vC,Omega] = fcn(vL,vR)
%#codegen

d= 0.235;

vC=0.5*(vL+vR);
Omega=(1/d)*(vR-vL);

== matlab function Qbot2_Full_Kinematics (No Gyro)/Qbot2_Kinematics (No Gyro)/Qbot2_Kinematics (Vf,W to x_dot,y_dot and psi_dot) ==
  data: vC input double; x_dot output double; Omega input double; y_dot output double; psi input double; psi_dot output double
function [x_dot,y_dot,psi_dot] = fcn(vC,Omega,psi)
%#codegen


x_dot=cos(psi)*vC;
y_dot=sin(psi)*vC;
psi_dot= Omega;

== matlab function Enabled Subsystem/MATLAB Function ==
  data: rgb_coords input double; X output double; depth_mm input double; Y output double; THETA output double
function [X, Y, THETA] = fcn(rgb_coords, depth_mm)
%#codegen

rgb_coords_x = 320 - rgb_coords(1);
%rgb_coords_y = rgb_coords(2);
X_offset_mm = 14;
%RGB_PX_COUNT_HORIZONTAL = 640;
%RGB_FOV_HORIZONTAL_DEG = 57;
%RGB_FOV_HORIZONTAL_RAD = 0.99483767363676785884650373803851;
% 0.00155443386505744977944766209069
RGB_DEG_PER_PX_HORIZONTAL = double(0.0015544);



THETA = 0;
X = double(depth_mm + X_offset_mm) / 1000;

% RGB camera not centered, so error changes with object distance
% I mean to say we are not currently correcting for this

Y = X * tan(rgb_coords_x * RGB_DEG_PER_PX_HORIZONTAL);
